simulink library "NbLibrary"  (Simulink 7.5)
settings: Solver=ode45  StartTime=0.0  StopTime=10.0  RelTol=1e-3
values from neighbouring files (symbols this model uses):
  asd = noiseAC(getProbeNum(opt,probename),:)    [OptickleFlexTF.m]    (also in nbAcquireData.m = interp1(f, sqrt(psd), freq, 'nearest', 0); nbLive.m = interp1(f, sqrt(psd), freq); optickleNoiseBlock.m; optickleNoiseBlock01.m)
settings Model: Creator=ccw  LastModifiedBy=controls

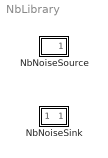
== system NbLibrary ==
  NbNoiseSink : Subsystem  Tag=NbNoiseSink  mask{dof='DOF'}
      mask prompts: dof "DOF name"
      settings: AttributesFormatString=%<Tag>
  NbNoiseSource : Subsystem  Tag=NbNoiseSource  mask{asd=asd}
      mask prompts: asd "Amplitude spectral density"
      settings: AttributesFormatString=%<Tag>

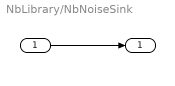
== system NbLibrary/NbNoiseSink ==
  " " : Inport
  "  " : Outport
  wires:
  " "/1 -> "  "/1

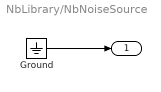
== system NbLibrary/NbNoiseSource ==
  Ground : Ground
  " " : Outport
  wires:
  Ground/1 -> " "/1
